simulink model "Casc_Filter_reva"  (Simulink 6.6)
settings: Solver=ode45  StartTime=0.0  StopTime=32768/sampling_freq  RelTol=1e-3
values from neighbouring files (symbols this model uses):
  filter_clk = sampling_freq*clk_mult    (= 375000000)    [Cascade_Taps_reva.m]    (also in Casecade_Taps.m)
  h_g = round(h_g*2^17)/2^17    [Cascade_Taps_reva.m]    (also in Casecade_Taps.m)
  h_k = round(h_k*2^17)/2^17    [Cascade_Taps_reva.m]    (also in Casecade_Taps.m)
  sampling_freq = 125e6    (= 125000000)    [Cascade_Taps_reva.m]    (also in Casecade_Taps.m)
undefined symbols (not defined in the file or in its folder): A, B, Fs, get, PCIN
libraries: xbsIndex_r4 x314, dspsnks4 x3, dspsrcs4 x2, simulink x2
(part 1 of 3)
settings Model: Creator=tbrimeye  LastModifiedBy=ericloew
settings DebuggingCC: SignalResolutionControl=TryResolveAllWithWarning  MultiTaskDSMMsg=warning  MultiTaskCondExecSysMsg=none
settings RTWCC: IncludeERTFirstTime=on

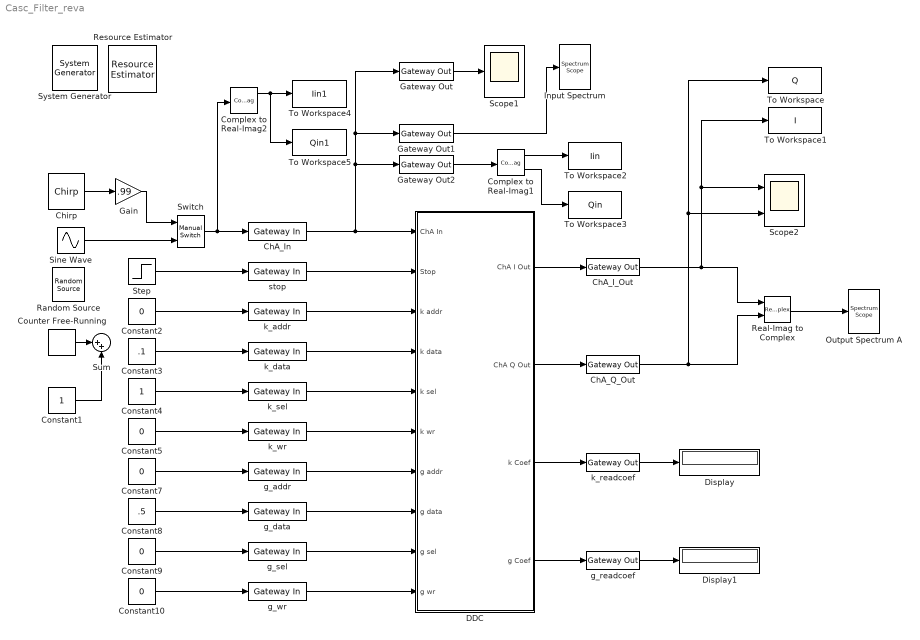
== system Casc_Filter_reva ==
  " System Generator" : xbsIndex_r4/ System Generator  Tag=genX  SystemSampleTime=-1  xilinxfamily=virtex4  part=xc4vsx55  speed=-10  package=ff1148  synthesis_tool=XST  directory=C:/GateFlow/7142_sig/4953_s142/xc4vsx55/Matlab/SysGen_Outputs  testbench=off  simulink_period=1/filter_clk  sysclk_period=(1/filter_clk)*1e9  incr_netlist=off  trim_vbits=Everywhere in SubSystem  dbl_ovrd=According to Block Masks  core_generation=According to Block Masks  run_coregen=off  deprecated_control=off  eval_field=0  block_type=sysgen
      settings: block_version=8.2
  ChA_I_Out : xbsIndex_r4/Gateway Out  hdl_port=on  timing_constraint=Data Rate  locs_specified=off  LOCs={}  block_type=gatewayout
      settings: infoedit="Gateway out block.  Converts Xilinx fixed point inputs into ouputs of type Simulink integer, double, or fixed point.<P><P>Hardware notes:  In hardware these blocks become top level output ports or are discarded, depending on how they are configured."  xl_area=[0 0 0 0 16 0 0]  block_version=8.2
  ChA_In : xbsIndex_r4/Gateway In  arith_type="Signed  (2's comp)"  n_bits=14  bin_pt=13  quantization="Round  (unbiased: +/- Inf)"  overflow=Saturate  period=1/sampling_freq  dbl_ovrd=off  timing_constraint=Data Rate  locs_specified=off  LOCs={}  block_type=gatewayin
      settings: infoedit="Gateway in block.  Converts inputs of type Simulink integer, double and fixed point to  Xilinx fixed point type.<P><P>Hardware notes:  In hardware these blocks become top level input ports."  xl_area=[0 0 0 0 14 0 0]  block_version=8.2
  ChA_Q_Out : xbsIndex_r4/Gateway Out  hdl_port=on  timing_constraint=Data Rate  locs_specified=off  LOCs={}  block_type=gatewayout
      settings: infoedit="Gateway out block.  Converts Xilinx fixed point inputs into ouputs of type Simulink integer, double, or fixed point.<P><P>Hardware notes:  In hardware these blocks become top level output ports or are discarded, depending on how they are configured."  xl_area=[0 0 0 0 16 0 0]  block_version=8.2
  Chirp : dspsrcs4/Chirp  sweep=Linear  mode=Unidirectional  f0=148.25e6  f1=164.25e6  t1=8192/sampling_freq  Tsweep=8192/sampling_freq  phase=pi/4  Ts=1/sampling_freq  spf=1  datatype=Double
  Complex to Real-Imag1 : ComplexToRealImag
  Complex to Real-Imag2 : ComplexToRealImag
  Constant1 : Constant
  Constant{2,5,7,9..10} (5 alike) : Constant  Value=0
  Constant3 : Constant  Value=.1
  Constant4 : Constant
  Constant8 : Constant  Value=.5
  Counter Free-Running : simulink/Sources/Counter Free-Running  SystemSampleTime=-1  NumBits=16  tsamp=1/sampling_freq
  DDC : Subsystem
  Display : Display
  Display1 : Display
  Gain : Gain  Gain=.99
  Gateway Out : xbsIndex_r4/Gateway Out  hdl_port=off  timing_constraint=None  locs_specified=off  LOCs={}  block_type=gatewayout
      settings: infoedit="Gateway out block.  Converts Xilinx fixed point inputs into ouputs of type Simulink integer, double, or fixed point.<P><P>Hardware notes:  In hardware these blocks become top level output ports or are discarded, depending on how they are configured."  block_version=8.2
  Gateway Out1 : xbsIndex_r4/Gateway Out  hdl_port=off  timing_constraint=None  locs_specified=off  LOCs={}  block_type=gatewayout
      settings: infoedit="Gateway out block.  Converts Xilinx fixed point inputs into ouputs of type Simulink integer, double, or fixed point.<P><P>Hardware notes:  In hardware these blocks become top level output ports or are discarded, depending on how they are configured."  block_version=8.2
  Gateway Out2 : xbsIndex_r4/Gateway Out  hdl_port=off  timing_constraint=None  locs_specified=off  LOCs={}  block_type=gatewayout
      settings: infoedit="Gateway out block.  Converts Xilinx fixed point inputs into ouputs of type Simulink integer, double, or fixed point.<P><P>Hardware notes:  In hardware these blocks become top level output ports or are discarded, depending on how they are configured."  block_version=8.2
  Input Spectrum : dspsnks4/Spectrum Scope  DialogController=dspdialog.SpectrumScope  DialogControllerArgs=DataTag2  SystemSampleTime=-1  ScopeProperties=on  Domain=Frequency  HorizSpan=1  UseBuffer=on  BufferSize=4096  Overlap=64  inpFftLenInherit=on  FFTlength=4096  numAvg=4  DisplayProperties=off  AxisGrid=on  Memory=off  FrameNumber=on  AxisLegend=off  AxisZoom=off  OpenScopeAtSimStart=on  OpenScopeImmediately=off  FigPos=get(0,'defaultfigureposition')  AxisProperties=off  XUnits=Hertz  XRange=[-Fs/2...Fs/2]  InheritXIncr=on  XIncr=1.0  XLabel=Samples  XLimit=Auto  YUnits=dB  XMax=1  XMin=0  YLabel=Magnitude-squared, dB  LineProperties=off  wintypeSpecScope=Boxcar  RsSpecScope=50  betaSpecScope=5  winsampSpecScope=Periodic
      settings: YMin=-38.4292198849576  YMax=29.4113653509126
  Output Spectrum A : dspsnks4/Spectrum Scope  DialogController=dspdialog.SpectrumScope  DialogControllerArgs=DataTag3  SystemSampleTime=-1  ScopeProperties=on  Domain=Frequency  HorizSpan=1  UseBuffer=on  BufferSize=1024  Overlap=64  inpFftLenInherit=on  FFTlength=1024  numAvg=1  DisplayProperties=off  AxisGrid=on  Memory=off  FrameNumber=on  AxisLegend=off  AxisZoom=off  OpenScopeAtSimStart=on  OpenScopeImmediately=off  FigPos=get(0,'defaultfigureposition')  AxisProperties=off  XUnits=Hertz  XRange=[-Fs/2...Fs/2]  InheritXIncr=on  XIncr=1.0  XLabel=Samples  XLimit=Auto  YUnits=dB  XMax=1  XMin=0  YLabel=Magnitude-squared, dB  LineProperties=off  wintypeSpecScope=Boxcar  RsSpecScope=50  betaSpecScope=5  winsampSpecScope=Symmetric
      settings: YMin=-135.913616439453  YMax=3.76850779494313
  Random Source : dspsrcs4/Random Source  SrcType=Uniform  NormMethod=Ziggurat  CltLength=12  MinVal=-1  MaxVal=1  MeanVal=0  VarVal=1  RepMode=Not repeatable  rawSeed=1  IsInherit=off  SampMode=Discrete  SampTime=1/sampling_freq  SampFrame=1  DataType=Double  OutComplex=Real
  Real-Imag to Complex : RealImagToComplex
  Resource Estimator : xbsIndex_r4/Resource Estimator  Tag=resEstTag  Slices=925  FFs=1405  BRAMs=7  LUTs=1104  IOBs=133  EBMs=14  TBUFs=0  xl_use_estimator_area=off  est_options=Post Map  xl_estimator_area=[1915 2342 0 3405 33 4 0]  block_type=resource_estimator
      settings: AttributesFormatString=Resource\nEstimator  block_version=8.2
  Scope1 : Scope
      settings: SaveName=ScopeData2
  Scope2 : Scope  NumInputPorts=2
      settings: YMin=-5~-5  YMax=5~5  SaveName=ScopeData4
  Sine Wave : Sin  Amplitude=.99  Frequency=2*pi*156.75e6  SampleTime=1/sampling_freq
  Step : Step  Time=00/filter_clk  Before=1  After=0  SampleTime=1/filter_clk
  Sum : Sum  Inputs=|++
  Switch : simulink/Signal Routing/Manual Switch  SystemSampleTime=-1  sw=1  action=0  varsize=off
  To Workspace : ToWorkspace  VariableName=Q  SampleTime=-1  SaveFormat=Array
  To Workspace1 : ToWorkspace  VariableName=I  SampleTime=-1  SaveFormat=Array
  To Workspace2 : ToWorkspace  VariableName=Iin  SampleTime=-1  SaveFormat=Array
  To Workspace3 : ToWorkspace  VariableName=Qin  SampleTime=-1  SaveFormat=Array
  To Workspace4 : ToWorkspace  VariableName=Iin1  SampleTime=-1  SaveFormat=Array
  To Workspace5 : ToWorkspace  VariableName=Qin1  SampleTime=-1  SaveFormat=Array
  g_addr : xbsIndex_r4/Gateway In  arith_type=Unsigned  n_bits=4  bin_pt=0  quantization="Round  (unbiased: +/- Inf)"  overflow=Saturate  period=1/sampling_freq  dbl_ovrd=off  timing_constraint=None  locs_specified=off  LOCs={}  block_type=gatewayin
      settings: infoedit="Gateway in block.  Converts inputs of type Simulink integer, double and fixed point to  Xilinx fixed point type.<P><P>Hardware notes:  In hardware these blocks become top level input ports."  xl_area=[0 0 0 0 4 0 0]  block_version=VER_STRING_GOES_HERE
  g_data : xbsIndex_r4/Gateway In  arith_type="Signed  (2's comp)"  n_bits=18  bin_pt=17  quantization="Round  (unbiased: +/- Inf)"  overflow=Saturate  period=1/sampling_freq  dbl_ovrd=off  timing_constraint=None  locs_specified=off  LOCs={}  block_type=gatewayin
      settings: infoedit="Gateway in block.  Converts inputs of type Simulink integer, double and fixed point to  Xilinx fixed point type.<P><P>Hardware notes:  In hardware these blocks become top level input ports."  xl_area=[0 0 0 0 18 0 0]  block_version=VER_STRING_GOES_HERE
  g_readcoef : xbsIndex_r4/Gateway Out  hdl_port=on  timing_constraint=Data Rate  locs_specified=off  LOCs={}  block_type=gatewayout
      settings: infoedit="Gateway out block.  Converts Xilinx fixed point inputs into ouputs of type Simulink integer, double, or fixed point.<P><P>Hardware notes:  In hardware these blocks become top level output ports or are discarded, depending on how they are configured."  xl_area=[0 0 0 0 18 0 0]  block_version=VER_STRING_GOES_HERE
  g_sel : xbsIndex_r4/Gateway In  arith_type=Unsigned  n_bits=2  bin_pt=0  quantization="Round  (unbiased: +/- Inf)"  overflow=Saturate  period=1/sampling_freq  dbl_ovrd=off  timing_constraint=None  locs_specified=off  LOCs={}  block_type=gatewayin
      settings: infoedit="Gateway in block.  Converts inputs of type Simulink integer, double and fixed point to  Xilinx fixed point type.<P><P>Hardware notes:  In hardware these blocks become top level input ports."  xl_area=[0 0 0 0 2 0 0]  block_version=VER_STRING_GOES_HERE
  g_wr : xbsIndex_r4/Gateway In  arith_type=Boolean  n_bits=4  bin_pt=0  quantization="Round  (unbiased: +/- Inf)"  overflow=Saturate  period=1/sampling_freq  dbl_ovrd=off  timing_constraint=None  locs_specified=off  LOCs={}  block_type=gatewayin
      settings: infoedit="Gateway in block.  Converts inputs of type Simulink integer, double and fixed point to  Xilinx fixed point type.<P><P>Hardware notes:  In hardware these blocks become top level input ports."  xl_area=[0 0 0 0 1 0 0]  block_version=VER_STRING_GOES_HERE
  k_addr : xbsIndex_r4/Gateway In  arith_type=Unsigned  n_bits=4  bin_pt=0  quantization="Round  (unbiased: +/- Inf)"  overflow=Saturate  period=1/sampling_freq  dbl_ovrd=off  timing_constraint=None  locs_specified=off  LOCs={}  block_type=gatewayin
      settings: infoedit="Gateway in block.  Converts inputs of type Simulink integer, double and fixed point to  Xilinx fixed point type.<P><P>Hardware notes:  In hardware these blocks become top level input ports."  xl_area=[0 0 0 0 4 0 0]  block_version=VER_STRING_GOES_HERE
  k_data : xbsIndex_r4/Gateway In  arith_type="Signed  (2's comp)"  n_bits=18  bin_pt=17  quantization="Round  (unbiased: +/- Inf)"  overflow=Saturate  period=1/sampling_freq  dbl_ovrd=off  timing_constraint=None  locs_specified=off  LOCs={}  block_type=gatewayin
      settings: infoedit="Gateway in block.  Converts inputs of type Simulink integer, double and fixed point to  Xilinx fixed point type.<P><P>Hardware notes:  In hardware these blocks become top level input ports."  xl_area=[0 0 0 0 18 0 0]  block_version=VER_STRING_GOES_HERE
  k_readcoef : xbsIndex_r4/Gateway Out  hdl_port=on  timing_constraint=Data Rate  locs_specified=off  LOCs={}  block_type=gatewayout
      settings: infoedit="Gateway out block.  Converts Xilinx fixed point inputs into ouputs of type Simulink integer, double, or fixed point.<P><P>Hardware notes:  In hardware these blocks become top level output ports or are discarded, depending on how they are configured."  xl_area=[0 0 0 0 18 0 0]  block_version=VER_STRING_GOES_HERE
  k_sel : xbsIndex_r4/Gateway In  arith_type=Unsigned  n_bits=3  bin_pt=0  quantization="Round  (unbiased: +/- Inf)"  overflow=Saturate  period=1/sampling_freq  dbl_ovrd=off  timing_constraint=None  locs_specified=off  LOCs={}  block_type=gatewayin
      settings: infoedit="Gateway in block.  Converts inputs of type Simulink integer, double and fixed point to  Xilinx fixed point type.<P><P>Hardware notes:  In hardware these blocks become top level input ports."  xl_area=[0 0 0 0 2 0 0]  block_version=VER_STRING_GOES_HERE
  k_wr : xbsIndex_r4/Gateway In  arith_type=Boolean  n_bits=4  bin_pt=0  quantization="Round  (unbiased: +/- Inf)"  overflow=Saturate  period=1/sampling_freq  dbl_ovrd=off  timing_constraint=None  locs_specified=off  LOCs={}  block_type=gatewayin
      settings: infoedit="Gateway in block.  Converts inputs of type Simulink integer, double and fixed point to  Xilinx fixed point type.<P><P>Hardware notes:  In hardware these blocks become top level input ports."  xl_area=[0 0 0 0 1 0 0]  block_version=VER_STRING_GOES_HERE
  stop : xbsIndex_r4/Gateway In  arith_type=Unsigned  n_bits=1  bin_pt=0  quantization="Round  (unbiased: +/- Inf)"  overflow=Saturate  period=1/sampling_freq  dbl_ovrd=off  timing_constraint=Data Rate  locs_specified=off  LOCs={}  block_type=gatewayin
      settings: infoedit="Gateway in block.  Converts inputs of type Simulink integer, double and fixed point to  Xilinx fixed point type.<P><P>Hardware notes:  In hardware these blocks become top level input ports."  xl_area=[0 0 0 0 1 0 0]  block_version=VER_STRING_GOES_HERE
  wires:
  Chirp/1 -> Gain/1
  ChA_In/1 -> DDC/1(ChA In), Gateway Out1/1, Gateway Out/1, Gateway Out2/1
  Real-Imag to Complex/1 -> Output Spectrum A/1
  Switch/1 -> ChA_In/1, Complex to Real-Imag2/1
  ChA_I_Out/1 -> Real-Imag to Complex/1, Scope2/1, To Workspace1/1
  ChA_Q_Out/1 -> Real-Imag to Complex/2, Scope2/2, To Workspace/1
  k_sel/1 -> DDC/5(k sel)
  k_addr/1 -> DDC/3(k addr)
  k_data/1 -> DDC/4(k data)
  k_wr/1 -> DDC/6(k wr)
  DDC/3(k Coef) -> k_readcoef/1
  Constant2/1 -> k_addr/1
  Constant3/1 -> k_data/1
  Constant4/1 -> k_sel/1
  Constant5/1 -> k_wr/1
  k_readcoef/1 -> Display/1
  g_readcoef/1 -> Display1/1
  DDC/4(g Coef) -> g_readcoef/1
  g_addr/1 -> DDC/7(g addr)
  g_data/1 -> DDC/8(g data)
  g_sel/1 -> DDC/9(g sel)
  g_wr/1 -> DDC/10(g wr)
  Constant7/1 -> g_addr/1
  Constant8/1 -> g_data/1
  Constant9/1 -> g_sel/1
  Constant10/1 -> g_wr/1
  DDC/1(ChA I Out) -> ChA_I_Out/1
  DDC/2(ChA Q Out) -> ChA_Q_Out/1
  stop/1 -> DDC/2(Stop)
  Gateway Out/1 -> Scope1/1
  Gateway Out1/1 -> Input Spectrum/1
  Gain/1 -> Switch/1
  Gateway Out2/1 -> Complex to Real-Imag1/1
  Complex to Real-Imag2/1 -> To Workspace4/1, To Workspace5/1
  Step/1 -> stop/1
  Counter Free-Running/1 -> Sum/1
  Constant1/1 -> Sum/2
  Complex to Real-Imag1/1 -> To Workspace2/1
  Complex to Real-Imag1/2 -> To Workspace3/1
  Sine Wave/1 -> Switch/2

== system Casc_Filter_reva/DDC ==
  ChA In : Inport
  Stop : Inport  Port=2
  k addr : Inport  Port=3
  k data : Inport  Port=4
  k sel : Inport  Port=5
  k wr : Inport  Port=6
  g addr : Inport  Port=7
  g data : Inport  Port=8
  g sel : Inport  Port=9
  g wr : Inport  Port=10
  Coefficients : Subsystem
  Count Generator : Subsystem
  DDC A : Subsystem
  Display : Display
  ChA I Out : Outport
  ChA Q Out : Outport  Port=2
  k Coef : Outport  Port=3
  g Coef : Outport  Port=4
  wires:
  Count Generator/1(Count) -> Coefficients/1(Counter), DDC A/1(Counter)
  Coefficients/1(k_Coef0) -> DDC A/4(k_Coef0)
  Coefficients/2(k_Coef1) -> DDC A/5(k_Coef1)
  Coefficients/3(k_Coef2) -> DDC A/6(k_Coef2)
  Coefficients/4(k_Coef3) -> DDC A/7(k_Coef3)
  Count Generator/2(Invert Count) -> DDC A/2(Counter Inv)
  Coefficients/5(g_Coef0) -> DDC A/12(g_Coef0), Display/1
  Coefficients/10(g_Coef1) -> DDC A/13(g_Coef1)
  Coefficients/11(g_Coef2) -> DDC A/14(g_Coef2)
  ChA In/1 -> DDC A/3(Data In Ch A)
  Stop/1 -> Coefficients/2(Stop), Count Generator/1(Reset)
  k addr/1 -> Coefficients/3(k_addr)
  k data/1 -> Coefficients/4(k_data)
  k sel/1 -> Coefficients/5(k_sel)
  k wr/1 -> Coefficients/6(k_wr)
  g addr/1 -> Coefficients/7(g_addr)
  g data/1 -> Coefficients/8(g_data)
  Coefficients/12(k_CoefRead) -> k Coef/1
  g sel/1 -> Coefficients/9(g_sel)
  g wr/1 -> Coefficients/10(g_wr)
  Coefficients/13(g_CoefRead) -> g Coef/1
  DDC A/1(I Out) -> ChA I Out/1
  DDC A/2(Q Out) -> ChA Q Out/1
  Coefficients/6(k_Coef4) -> DDC A/8(k_Coef4)
  Coefficients/7(k_Coef5) -> DDC A/9(k_Coef5)
  Coefficients/8(k_Coef6) -> DDC A/10(k_Coef6)
  Coefficients/9(k_Coef7) -> DDC A/11(k_Coef7)

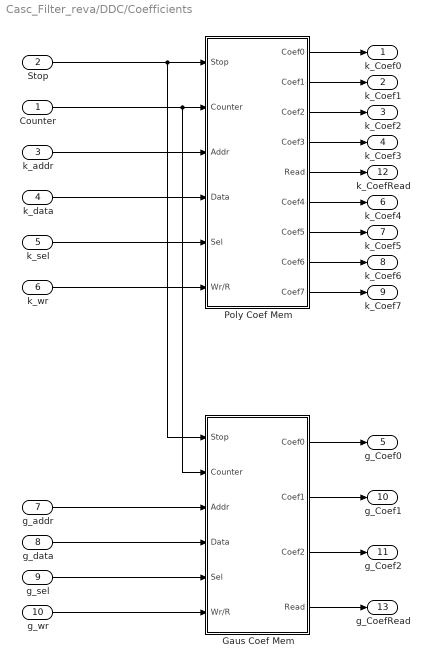
== system Casc_Filter_reva/DDC/Coefficients ==
  Counter : Inport
  Stop : Inport  Port=2
  k_addr : Inport  Port=3
  k_data : Inport  Port=4
  k_sel : Inport  Port=5
  k_wr : Inport  Port=6
  g_addr : Inport  Port=7
  g_data : Inport  Port=8
  g_sel : Inport  Port=9
  g_wr : Inport  Port=10
  Gaus Coef Mem : Subsystem
  Poly Coef Mem : Subsystem
  k_Coef0 : Outport
  k_Coef1 : Outport  Port=2
  k_Coef2 : Outport  Port=3
  k_Coef3 : Outport  Port=4
  g_Coef0 : Outport  Port=5
  k_Coef4 : Outport  Port=6
  k_Coef5 : Outport  Port=7
  k_Coef6 : Outport  Port=8
  k_Coef7 : Outport  Port=9
  g_Coef1 : Outport  Port=10
  g_Coef2 : Outport  Port=11
  k_CoefRead : Outport  Port=12
  g_CoefRead : Outport  Port=13
  wires:
  Stop/1 -> Gaus Coef Mem/1(Stop), Poly Coef Mem/1(Stop)
  Counter/1 -> Poly Coef Mem/2(Counter), Gaus Coef Mem/2(Counter)
  Poly Coef Mem/1(Coef0) -> k_Coef0/1
  Poly Coef Mem/2(Coef1) -> k_Coef1/1
  k_addr/1 -> Poly Coef Mem/3(Addr)
  Poly Coef Mem/3(Coef2) -> k_Coef2/1
  k_data/1 -> Poly Coef Mem/4(Data)
  Poly Coef Mem/4(Coef3) -> k_Coef3/1
  k_sel/1 -> Poly Coef Mem/5(Sel)
  Poly Coef Mem/5(Read) -> k_CoefRead/1
  k_wr/1 -> Poly Coef Mem/6(Wr/R)
  Gaus Coef Mem/1(Coef0) -> g_Coef0/1
  Gaus Coef Mem/2(Coef1) -> g_Coef1/1
  g_addr/1 -> Gaus Coef Mem/3(Addr)
  g_data/1 -> Gaus Coef Mem/4(Data)
  Gaus Coef Mem/3(Coef2) -> g_Coef2/1
  g_sel/1 -> Gaus Coef Mem/5(Sel)
  Gaus Coef Mem/4(Read) -> g_CoefRead/1
  g_wr/1 -> Gaus Coef Mem/6(Wr/R)
  Poly Coef Mem/6(Coef4) -> k_Coef4/1
  Poly Coef Mem/7(Coef5) -> k_Coef5/1
  Poly Coef Mem/8(Coef6) -> k_Coef6/1
  Poly Coef Mem/9(Coef7) -> k_Coef7/1

== system Casc_Filter_reva/DDC/Count Generator ==
  Reset : Inport
  AddSub : xbsIndex_r4/AddSub  mode=Subtraction  use_carryin=off  use_carryout=off  en=off  latency=0  precision=User Defined  arith_type=Unsigned  n_bits=3  bin_pt=0  quantization=Truncate  overflow=Wrap  dbl_ovrd=off  use_behavioral_HDL=off  pipelined=off  use_rpm=on  block_type=addsub
      settings: block_version=9.2.01
  Constant : xbsIndex_r4/Constant  arith_type=Unsigned  const=7  n_bits=4  bin_pt=0  explicit_period=off  period=1  equ=P=C  opselect=C  inp2=PCIN>>17  opr=+  inp1=P  carry=CIN  dbl_ovrd=off  block_type=constant
      settings: block_version=9.2.01
  Convert : xbsIndex_r4/Convert  arith_type=Boolean  n_bits=16  bin_pt=14  quantization=Truncate  overflow=Wrap  latency=0  dbl_ovrd=off  pipeline=off  block_type=convert
      settings: block_version=9.2.01
  Counter : xbsIndex_r4/Counter  cnt_type=Count Limited  cnt_to=7  operation=Up  start_count=0  cnt_by_val=1  arith_type=Unsigned  n_bits=3  bin_pt=0  load_pin=off  rst=on  en=off  explicit_period=on  period=1/filter_clk  dbl_ovrd=off  use_behavioral_HDL=off  use_rpm=off  block_type=counter
      settings: block_version=8.2
  Count : Outport
  Invert Count : Outport  Port=2
  wires:
  Counter/1 -> AddSub/2, Count/1
  Constant/1 -> AddSub/1
  Convert/1 -> Counter/1
  Reset/1 -> Convert/1
  AddSub/1 -> Invert Count/1

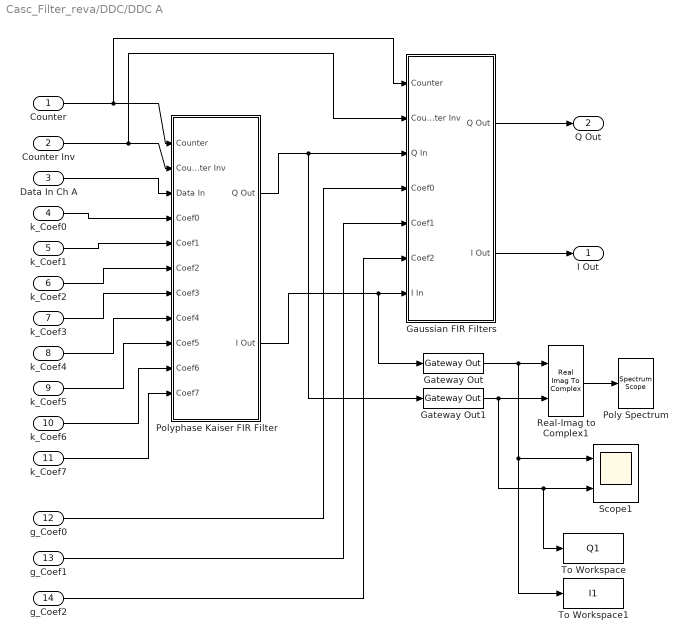
== system Casc_Filter_reva/DDC/DDC A ==
  Counter : Inport
  Counter Inv : Inport  Port=2
  Data In Ch A : Inport  Port=3
  k_Coef0 : Inport  Port=4
  k_Coef1 : Inport  Port=5
  k_Coef2 : Inport  Port=6
  k_Coef3 : Inport  Port=7
  k_Coef4 : Inport  Port=8
  k_Coef5 : Inport  Port=9
  k_Coef6 : Inport  Port=10
  k_Coef7 : Inport  Port=11
  g_Coef0 : Inport  Port=12
  g_Coef1 : Inport  Port=13
  g_Coef2 : Inport  Port=14
  Gateway Out : xbsIndex_r4/Gateway Out  hdl_port=off  timing_constraint=None  locs_specified=off  LOCs={}  block_type=gatewayout
      settings: infoedit="Gateway out block.  Converts Xilinx fixed point inputs into ouputs of type Simulink integer, double, or fixed point.<P><P>Hardware notes:  In hardware these blocks become top level output ports or are discarded, depending on how they are configured."  block_version=8.2
  Gateway Out1 : xbsIndex_r4/Gateway Out  hdl_port=off  timing_constraint=None  locs_specified=off  LOCs={}  block_type=gatewayout
      settings: infoedit="Gateway out block.  Converts Xilinx fixed point inputs into ouputs of type Simulink integer, double, or fixed point.<P><P>Hardware notes:  In hardware these blocks become top level output ports or are discarded, depending on how they are configured."  block_version=8.2
  Gaussian FIR Filters : Subsystem
  Poly Spectrum : dspsnks4/Spectrum Scope  DialogController=dspdialog.SpectrumScope  DialogControllerArgs=DataTag1  SystemSampleTime=-1  ScopeProperties=on  Domain=Frequency  HorizSpan=1  UseBuffer=on  BufferSize=1024  Overlap=64  inpFftLenInherit=on  FFTlength=1024  numAvg=1  DisplayProperties=off  AxisGrid=on  Memory=off  FrameNumber=on  AxisLegend=off  AxisZoom=off  OpenScopeAtSimStart=on  OpenScopeImmediately=off  FigPos=get(0,'defaultfigureposition')  AxisProperties=off  XUnits=Hertz  XRange=[-Fs/2...Fs/2]  InheritXIncr=on  XIncr=1.0  XLabel=Samples  XLimit=Auto  YUnits=dB  XMax=1  XMin=0  YLabel=Magnitude-squared, dB  LineProperties=off  wintypeSpecScope=Boxcar  RsSpecScope=50  betaSpecScope=5  winsampSpecScope=Periodic
      settings: YMin=-87.1539985326234  YMax=2.74033893845064
  Polyphase Kaiser FIR Filter : Subsystem
  Real-Imag to Complex1 : RealImagToComplex
  Scope1 : Scope  NumInputPorts=2
      settings: YMin=-5~-5  YMax=5~5  SaveName=ScopeData3
  To Workspace : ToWorkspace  VariableName=Q1  SampleTime=-1  SaveFormat=Array
  To Workspace1 : ToWorkspace  VariableName=I1  SampleTime=-1  SaveFormat=Array
  I Out : Outport
  Q Out : Outport  Port=2
  wires:
  Counter Inv/1 -> Polyphase Kaiser FIR Filter/2(Counter Inv), Gaussian FIR Filters/2(Counter Inv)
  Real-Imag to Complex1/1 -> Poly Spectrum/1
  Counter/1 -> Polyphase Kaiser FIR Filter/1(Counter), Gaussian FIR Filters/1(Counter)
  Gaussian FIR Filters/1(Q Out) -> Q Out/1
  Data In Ch A/1 -> Polyphase Kaiser FIR Filter/3(Data In)
  k_Coef0/1 -> Polyphase Kaiser FIR Filter/4(Coef0)
  Gaussian FIR Filters/2(I Out) -> I Out/1
  k_Coef1/1 -> Polyphase Kaiser FIR Filter/5(Coef1)
  k_Coef2/1 -> Polyphase Kaiser FIR Filter/6(Coef2)
  Polyphase Kaiser FIR Filter/1(Q Out) -> Gaussian FIR Filters/3(Q In), Gateway Out1/1
  Polyphase Kaiser FIR Filter/2(I Out) -> Gaussian FIR Filters/7(I In), Gateway Out/1
  g_Coef0/1 -> Gaussian FIR Filters/4(Coef0)
  g_Coef1/1 -> Gaussian FIR Filters/5(Coef1)
  g_Coef2/1 -> Gaussian FIR Filters/6(Coef2)
  Gateway Out/1 -> Real-Imag to Complex1/1, Scope1/1, To Workspace1/1
  Gateway Out1/1 -> Real-Imag to Complex1/2, To Workspace/1, Scope1/2
  k_Coef4/1 -> Polyphase Kaiser FIR Filter/8(Coef4)
  k_Coef6/1 -> Polyphase Kaiser FIR Filter/10(Coef6)
  k_Coef7/1 -> Polyphase Kaiser FIR Filter/11(Coef7)
  k_Coef3/1 -> Polyphase Kaiser FIR Filter/7(Coef3)
  k_Coef5/1 -> Polyphase Kaiser FIR Filter/9(Coef5)

== system Casc_Filter_reva/DDC/Coefficients/Gaus Coef Mem ==
  Stop : Inport
  Counter : Inport  Port=2
  Addr : Inport  Port=3
  Data : Inport  Port=4
  Sel : Inport  Port=5
  Wr/R : Inport  Port=6
  Mux : xbsIndex_r4/Mux  inputs=2  en=off  latency=1  precision=Full  arith_type=Unsigned  n_bits=16  bin_pt=14  quantization=Truncate  overflow=Wrap  dbl_ovrd=off  block_type=mux
      settings: xl_area=[2 0 0 4 0 0 0]  block_version=VER_STRING_GOES_HERE
  Mux1 : xbsIndex_r4/Mux  inputs=3  en=on  latency=1  precision=Full  arith_type=Unsigned  n_bits=16  bin_pt=14  quantization=Truncate  overflow=Wrap  dbl_ovrd=off  block_type=mux
      settings: xl_area=[18 18 0 36 0 0 0]  block_version=VER_STRING_GOES_HERE
  Select Decoder : Subsystem
  Single Port RAM : xbsIndex_r4/Single Port RAM  depth=16  initVector=[h_g(1:8),0,0,0,0,0,0,0,0]  distributed_mem=Block RAM  write_mode=No Read On Write  rst=off  init_reg=0  en=off  latency=7  dbl_ovrd=off  optimize=Area  use_rpm=off  block_type=spram
      settings: xl_area=[18 0 0 36 0 0 0]  block_version=8.2
  Single Port RAM1 : xbsIndex_r4/Single Port RAM  depth=16  initVector=[h_g(9:16),0,0,0,0,0,0,0,0]  distributed_mem=Block RAM  write_mode=No Read On Write  rst=off  init_reg=0  en=off  latency=7  dbl_ovrd=off  optimize=Area  use_rpm=off  block_type=spram
      settings: xl_area=[18 0 0 36 0 0 0]  block_version=8.2
  Single Port RAM2 : xbsIndex_r4/Single Port RAM  depth=16  initVector=[h_g(17:24),0,0,0,0,0,0,0,0]  distributed_mem=Block RAM  write_mode=No Read On Write  rst=off  init_reg=0  en=off  latency=7  dbl_ovrd=off  optimize=Area  use_rpm=off  block_type=spram
      settings: xl_area=[18 0 0 36 0 0 0]  block_version=8.2
  Coef0 : Outport
  Coef1 : Outport  Port=2
  Coef2 : Outport  Port=3
  Read : Outport  Port=4
  wires:
  Data/1 -> Single Port RAM1/2, Single Port RAM2/2, Single Port RAM/2
  Single Port RAM/1 -> Mux1/2, Coef0/1
  Single Port RAM1/1 -> Mux1/3, Coef1/1
  Single Port RAM2/1 -> Mux1/4, Coef2/1
  Stop/1 -> Mux/1, Select Decoder/1(Run/Stop)
  Mux/1 -> Single Port RAM/1, Single Port RAM1/1, Single Port RAM2/1
  Mux1/1 -> Read/1
  Counter/1 -> Mux/2
  Addr/1 -> Mux/3
  Sel/1 -> Select Decoder/3(Sel), Mux1/1
  Select Decoder/2(Wr0) -> Single Port RAM/3
  Select Decoder/3(Wr1) -> Single Port RAM1/3
  Select Decoder/4(Wr2) -> Single Port RAM2/3
  Wr/R/1 -> Select Decoder/2(Wr/R)
  Select Decoder/1(R_En) -> Mux1/5

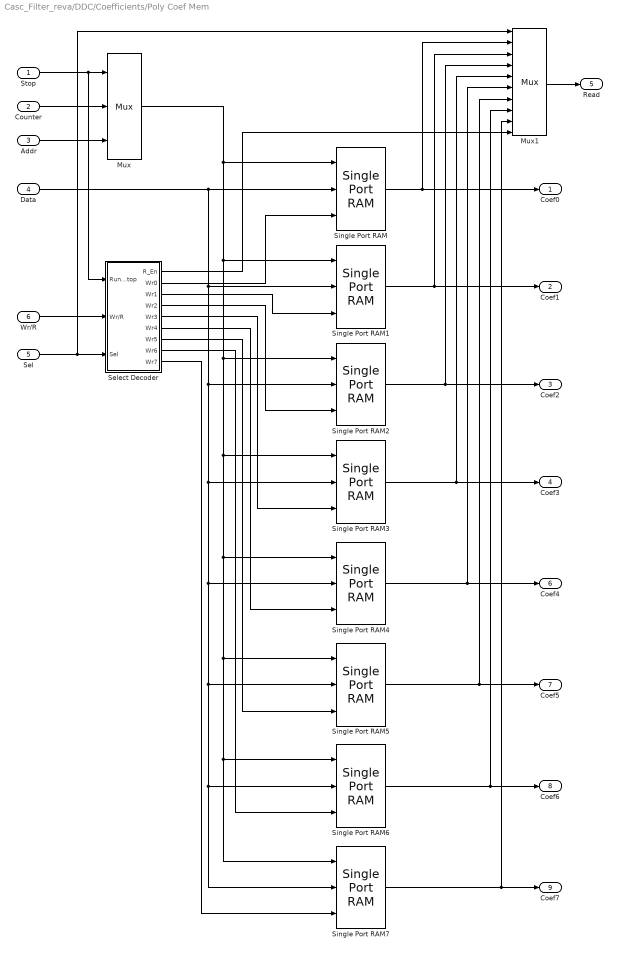
== system Casc_Filter_reva/DDC/Coefficients/Poly Coef Mem ==
  Stop : Inport
  Counter : Inport  Port=2
  Addr : Inport  Port=3
  Data : Inport  Port=4
  Sel : Inport  Port=5
  Wr/R : Inport  Port=6
  Mux : xbsIndex_r4/Mux  inputs=2  en=off  latency=1  precision=Full  arith_type=Unsigned  n_bits=16  bin_pt=14  quantization=Truncate  overflow=Wrap  dbl_ovrd=off  block_type=mux
      settings: xl_area=[2 0 0 4 0 0 0]  block_version=VER_STRING_GOES_HERE
  Mux1 : xbsIndex_r4/Mux  inputs=8  en=on  latency=1  precision=Full  arith_type=Unsigned  n_bits=16  bin_pt=14  quantization=Truncate  overflow=Wrap  dbl_ovrd=off  block_type=mux
      settings: xl_area=[18 18 0 36 0 0 0]  block_version=VER_STRING_GOES_HERE
  Select Decoder : Subsystem
  Single Port RAM : xbsIndex_r4/Single Port RAM  depth=16  initVector=[h_k(1:8:64),0,0,0,0,0,0,0,0]  distributed_mem=Block RAM  write_mode=No Read On Write  rst=off  init_reg=0  en=off  latency=7  dbl_ovrd=off  optimize=Area  use_rpm=off  block_type=spram
      settings: xl_area=[18 0 0 36 0 0 0]  block_version=8.2
  Single Port RAM1 : xbsIndex_r4/Single Port RAM  depth=16  initVector=[h_k(2:8:64),0,0,0,0,0,0,0,0]  distributed_mem=Block RAM  write_mode=No Read On Write  rst=off  init_reg=0  en=off  latency=7  dbl_ovrd=off  optimize=Area  use_rpm=off  block_type=spram
      settings: xl_area=[18 0 0 36 0 0 0]  block_version=8.2
  Single Port RAM2 : xbsIndex_r4/Single Port RAM  depth=16  initVector=[h_k(3:8:64),0,0,0,0,0,0,0,0]  distributed_mem=Block RAM  write_mode=No Read On Write  rst=off  init_reg=0  en=off  latency=7  dbl_ovrd=off  optimize=Area  use_rpm=off  block_type=spram
      settings: xl_area=[18 0 0 36 0 0 0]  block_version=8.2
  Single Port RAM3 : xbsIndex_r4/Single Port RAM  depth=16  initVector=[h_k(4:8:64),0,0,0,0,0,0,0,0]  distributed_mem=Block RAM  write_mode=No Read On Write  rst=off  init_reg=0  en=off  latency=7  dbl_ovrd=off  optimize=Area  use_rpm=off  block_type=spram
      settings: xl_area=[18 0 0 36 0 0 0]  block_version=8.2
  Single Port RAM4 : xbsIndex_r4/Single Port RAM  depth=16  initVector=[h_k(5:8:64),0,0,0,0,0,0,0,0]  distributed_mem=Block RAM  write_mode=No Read On Write  rst=off  init_reg=0  en=off  latency=7  dbl_ovrd=off  optimize=Area  use_rpm=off  block_type=spram
      settings: xl_area=[18 0 0 36 0 0 0]  block_version=8.2
  Single Port RAM5 : xbsIndex_r4/Single Port RAM  depth=16  initVector=[h_k(6:8:64),0,0,0,0,0,0,0,0]  distributed_mem=Block RAM  write_mode=No Read On Write  rst=off  init_reg=0  en=off  latency=7  dbl_ovrd=off  optimize=Area  use_rpm=off  block_type=spram
      settings: xl_area=[18 0 0 36 0 0 0]  block_version=8.2
  Single Port RAM6 : xbsIndex_r4/Single Port RAM  depth=16  initVector=[h_k(7:8:64),0,0,0,0,0,0,0,0]  distributed_mem=Block RAM  write_mode=No Read On Write  rst=off  init_reg=0  en=off  latency=7  dbl_ovrd=off  optimize=Area  use_rpm=off  block_type=spram
      settings: xl_area=[18 0 0 36 0 0 0]  block_version=8.2
  Single Port RAM7 : xbsIndex_r4/Single Port RAM  depth=16  initVector=[h_k(8:8:64),0,0,0,0,0,0,0,0]  distributed_mem=Block RAM  write_mode=No Read On Write  rst=off  init_reg=0  en=off  latency=7  dbl_ovrd=off  optimize=Area  use_rpm=off  block_type=spram
      settings: xl_area=[18 0 0 36 0 0 0]  block_version=8.2
  Coef0 : Outport
  Coef1 : Outport  Port=2
  Coef2 : Outport  Port=3
  Coef3 : Outport  Port=4
  Read : Outport  Port=5
  Coef4 : Outport  Port=6
  Coef5 : Outport  Port=7
  Coef6 : Outport  Port=8
  Coef7 : Outport  Port=9
  wires:
  Data/1 -> Single Port RAM2/2, Single Port RAM3/2, Single Port RAM4/2, Single Port RAM5/2, Single Port RAM6/2, Single Port RAM7/2, Single Port RAM1/2, Single Port RAM/2
  Single Port RAM/1 -> Mux1/2, Coef0/1
  Single Port RAM1/1 -> Mux1/3, Coef1/1
  Single Port RAM2/1 -> Mux1/4, Coef2/1
  Single Port RAM3/1 -> Mux1/5, Coef3/1
  Stop/1 -> Mux/1, Select Decoder/1(Run/Stop)
  Mux/1 -> Single Port RAM1/1, Single Port RAM2/1, Single Port RAM3/1, Single Port RAM4/1, Single Port RAM5/1, Single Port RAM6/1, Single Port RAM7/1, Single Port RAM/1
  Mux1/1 -> Read/1
  Counter/1 -> Mux/2
  Addr/1 -> Mux/3
  Sel/1 -> Select Decoder/3(Sel), Mux1/1
  Wr/R/1 -> Select Decoder/2(Wr/R)
  Select Decoder/2(Wr0) -> Single Port RAM/3
  Select Decoder/3(Wr1) -> Single Port RAM1/3
  Select Decoder/4(Wr2) -> Single Port RAM2/3
  Select Decoder/5(Wr3) -> Single Port RAM3/3
  Select Decoder/1(R_En) -> Mux1/10
  Single Port RAM4/1 -> Coef4/1, Mux1/6
  Single Port RAM5/1 -> Coef5/1, Mux1/7
  Single Port RAM6/1 -> Coef6/1, Mux1/8
  Single Port RAM7/1 -> Coef7/1, Mux1/9
  Select Decoder/6(Wr4) -> Single Port RAM4/3
  Select Decoder/7(Wr5) -> Single Port RAM5/3
  Select Decoder/8(Wr6) -> Single Port RAM6/3
  Select Decoder/9(Wr7) -> Single Port RAM7/3

== system Casc_Filter_reva/DDC/DDC A/Gaussian FIR Filters ==
  Counter : Inport
  Counter Inv : Inport  Port=2
  Q In : Inport  Port=3
  Coef0 : Inport  Port=4
  Coef1 : Inport  Port=5
  Coef2 : Inport  Port=6
  I In : Inport  Port=7
  Gaussian FIR Filter : Subsystem
  Gaussian FIR Filter1 : Subsystem
  Q Out : Outport
  I Out : Outport  Port=2
  wires:
  Counter/1 -> Gaussian FIR Filter/1(Counter), Gaussian FIR Filter1/1(Counter)
  Counter Inv/1 -> Gaussian FIR Filter/2(Counter Inv), Gaussian FIR Filter1/2(Counter Inv)
  Q In/1 -> Gaussian FIR Filter/3(Data In)
  I In/1 -> Gaussian FIR Filter1/3(Data In)
  Gaussian FIR Filter/1(Data Out) -> Q Out/1
  Gaussian FIR Filter1/1(Data Out) -> I Out/1
  Coef0/1 -> Gaussian FIR Filter/4(Coef0), Gaussian FIR Filter1/4(Coef0)
  Coef1/1 -> Gaussian FIR Filter/5(Coef1), Gaussian FIR Filter1/5(Coef1)
  Coef2/1 -> Gaussian FIR Filter/6(Coef2), Gaussian FIR Filter1/6(Coef2)

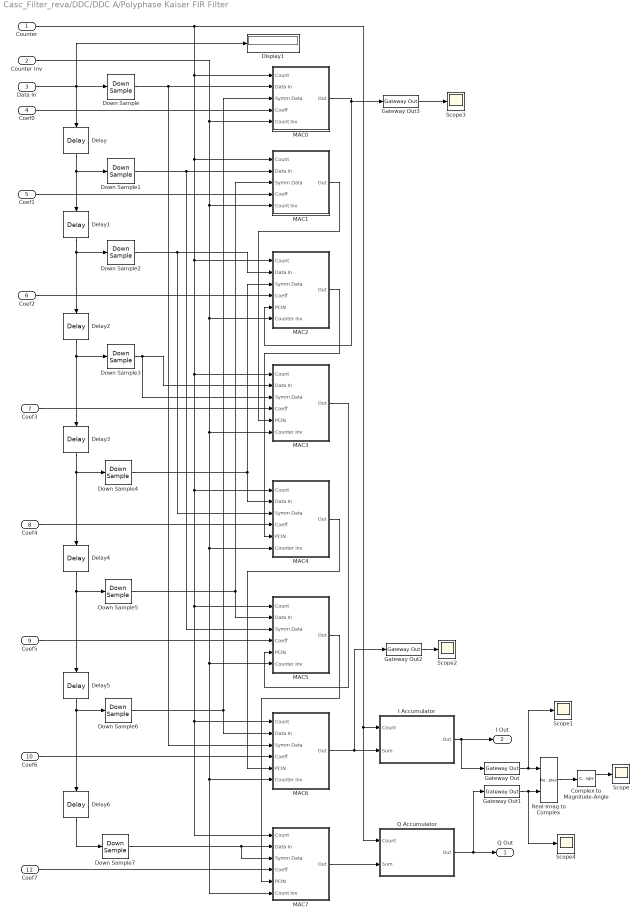
== system Casc_Filter_reva/DDC/DDC A/Polyphase Kaiser FIR Filter ==
  Counter : Inport
  Counter Inv : Inport  Port=2
  Data In : Inport  Port=3
  Coef0 : Inport  Port=4
  Coef1 : Inport  Port=5
  Coef2 : Inport  Port=6
  Coef3 : Inport  Port=7
  Coef4 : Inport  Port=8
  Coef5 : Inport  Port=9
  Coef6 : Inport  Port=10
  Coef7 : Inport  Port=11
  Complex to Magnitude-Angle : ComplexToMagnitudeAngle
  Delay{,1..6} (7 alike) : xbsIndex_r4/Delay  Orientation=down  en=off  latency=1  dbl_ovrd=off  reg_retiming=off  block_type=delay
      settings: infoedit=Hardware notes: A delay line is a chain, each link of which is an SRL16 followed by a flip-flop. If register retiming is enabled, the delay line is a chain of flip-flops.  block_version=8.2
  Display1 : Display
  Down Sample{,1..7} (8 alike) : xbsIndex_r4/Down Sample  sample_ratio=8  sample_phase="Last Value of Frame  (most efficient)"  en=off  latency=1  dbl_ovrd=off  block_type=dsamp
      settings: block_version=8.2
  Gateway Out{,1..3} (4 alike) : xbsIndex_r4/Gateway Out  hdl_port=off  timing_constraint=None  locs_specified=off  LOCs={}  block_type=gatewayout
      settings: infoedit="Gateway out block.  Converts Xilinx fixed point inputs into ouputs of type Simulink integer, double, or fixed point.<P><P>Hardware notes:  In hardware these blocks become top level output ports or are discarded, depending on how they are configured."  block_version=8.2
  I Accumulator : Subsystem
  MAC0 : Subsystem
  MAC1 : Subsystem
  MAC2 : Subsystem
  MAC3 : Subsystem
  MAC4 : Subsystem
  MAC5 : Subsystem
  MAC6 : Subsystem
  MAC7 : Subsystem
  Q Accumulator : Subsystem
  Real-Imag to Complex : RealImagToComplex
  Scope{,1..4} (5 alike) : Scope
      Scope2 settings: SaveName=ScopeData5
      Scope3 settings: SaveName=ScopeData6
      Scope4 settings: SaveName=ScopeData7
  Q Out : Outport
  I Out : Outport  Port=2
  wires:
  Coef7/1 -> MAC7/4(Coeff)
  Coef6/1 -> MAC6/4(Coeff)
  Coef5/1 -> MAC5/4(Coeff)
  Coef4/1 -> MAC4/4(Coeff)
  MAC5/1(Out) -> MAC7/5(PCIN)
  Down Sample7/1 -> MAC7/2(Data In), MAC7/3(Symm Data)
  MAC4/1(Out) -> MAC6/5(PCIN)
  Down Sample/1 -> MAC0/2(Data In), MAC6/3(Symm Data)
  Down Sample1/1 -> MAC1/2(Data In), MAC5/3(Symm Data)
  MAC3/1(Out) -> MAC5/5(PCIN)
  MAC2/1(Out) -> MAC4/5(PCIN)
  MAC1/1(Out) -> MAC3/5(PCIN)
  Down Sample3/1 -> MAC3/2(Data In), MAC3/3(Symm Data)
  Coef3/1 -> MAC3/4(Coeff)
  Coef2/1 -> MAC2/4(Coeff)
  MAC0/1(Out) -> MAC2/5(PCIN), Gateway Out3/1
  Down Sample2/1 -> MAC2/2(Data In), MAC4/3(Symm Data)
  Down Sample4/1 -> MAC2/3(Symm Data), MAC4/2(Data In)
  Down Sample5/1 -> MAC5/2(Data In), MAC1/3(Symm Data)
  Down Sample6/1 -> MAC0/3(Symm Data), MAC6/2(Data In)
  Delay6/1 -> Down Sample7/1
  Delay5/1 -> Down Sample6/1, Delay6/1
  Delay4/1 -> Down Sample5/1, Delay5/1
  Delay3/1 -> Down Sample4/1, Delay4/1
  Gateway Out1/1 -> Real-Imag to Complex/2, Scope4/1
  Gateway Out/1 -> Real-Imag to Complex/1, Scope1/1
  Complex to Magnitude-Angle/1 -> Scope/1
  Real-Imag to Complex/1 -> Complex to Magnitude-Angle/1
  Counter Inv/1 -> MAC1/5(Count Inv), MAC2/6(Counter Inv), MAC4/6(Counter Inv), MAC6/6(Counter Inv), MAC7/6(Count Inv), MAC5/6(Counter Inv), MAC3/6(Counter Inv), MAC0/5(Count Inv)
  MAC7/1(Out) -> Q Accumulator/2(Sum)
  MAC6/1(Out) -> I Accumulator/2(Sum), Gateway Out2/1
  Q Accumulator/1(Out) -> Q Out/1, Gateway Out1/1
  Counter/1 -> MAC1/1(Count), MAC2/1(Count), MAC3/1(Count), MAC4/1(Count), MAC7/1(Count), MAC6/1(Count), MAC5/1(Count), MAC0/1(Count), Q Accumulator/1(Count), I Accumulator/1(Count)
  I Accumulator/1(Out) -> I Out/1, Gateway Out/1
  Coef1/1 -> MAC1/4(Coeff)
  Coef0/1 -> MAC0/4(Coeff)
  Delay2/1 -> Down Sample3/1, Delay3/1
  Delay1/1 -> Down Sample2/1, Delay2/1
  Delay/1 -> Down Sample1/1, Delay1/1
  Data In/1 -> Down Sample/1, Delay/1, Display1/1
  Gateway Out2/1 -> Scope2/1
  Gateway Out3/1 -> Scope3/1

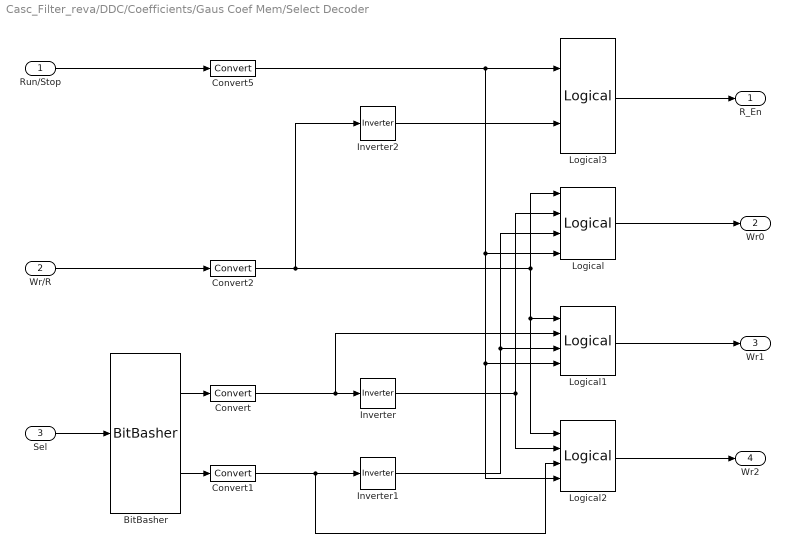
== system Casc_Filter_reva/DDC/Coefficients/Gaus Coef Mem/Select Decoder ==
  Run/Stop : Inport
  Wr/R : Inport  Port=2
  Sel : Inport  Port=3
  BitBasher : xbsIndex_r4/BitBasher  bitexpr=|  display_expr=off  sr_1=1  arith_type1=Unsigned  bin_pt1=0  sr_2=2  arith_type2=Unsigned  bin_pt2=0  sr_3=3  arith_type3=Unsigned  bin_pt3=0  sr_4=4  arith_type4=Unsigned  bin_pt4=0  dbl_ovrd=off  block_type=bitbasher
      | <html><head><meta name="qrichtext" content="1" /></head><body style="font-size:8pt;font-family:MS Shell Dlg">
      | <p>Sel0={Sel[0]}<br />Sel1={Sel[1]}<br /></p>
      | </body></html>
      settings: infoedit="Allows      extraction, concatenation and augmentation of bits"  block_version=VER_STRING_GOES_HERE
  Convert{,1..2,5} (4 alike) : xbsIndex_r4/Convert  arith_type=Boolean  n_bits=16  bin_pt=14  quantization=Truncate  overflow=Wrap  latency=0  dbl_ovrd=off  pipeline=off  block_type=convert
      settings: xl_area=[0 0 0 0 0 0 0]  block_version=VER_STRING_GOES_HERE
  Inverter : xbsIndex_r4/Inverter  en=off  latency=0  dbl_ovrd=off  block_type=inv
      settings: block_version=VER_STRING_GOES_HERE
  Inverter1 : xbsIndex_r4/Inverter  en=off  latency=0  dbl_ovrd=off  block_type=inv
      settings: block_version=VER_STRING_GOES_HERE
  Inverter2 : xbsIndex_r4/Inverter  en=off  latency=0  dbl_ovrd=off  block_type=inv
      settings: block_version=VER_STRING_GOES_HERE
  Logical : xbsIndex_r4/Logical  logical_function=AND  inputs=4  en=off  latency=0  precision=Full  arith_type=Unsigned  n_bits=16  bin_pt=0  align_bp=on  dbl_ovrd=off  block_type=logical
      settings: block_version=VER_STRING_GOES_HERE
  Logical1 : xbsIndex_r4/Logical  logical_function=AND  inputs=4  en=off  latency=0  precision=Full  arith_type=Unsigned  n_bits=16  bin_pt=0  align_bp=on  dbl_ovrd=off  block_type=logical
      settings: block_version=VER_STRING_GOES_HERE
  Logical2 : xbsIndex_r4/Logical  logical_function=AND  inputs=4  en=off  latency=0  precision=Full  arith_type=Unsigned  n_bits=16  bin_pt=0  align_bp=on  dbl_ovrd=off  block_type=logical
      settings: block_version=VER_STRING_GOES_HERE
  Logical3 : xbsIndex_r4/Logical  logical_function=AND  inputs=2  en=off  latency=0  precision=Full  arith_type=Unsigned  n_bits=16  bin_pt=0  align_bp=on  dbl_ovrd=off  block_type=logical
      settings: block_version=VER_STRING_GOES_HERE
  R_En : Outport
  Wr0 : Outport  Port=2
  Wr1 : Outport  Port=3
  Wr2 : Outport  Port=4
  wires:
  BitBasher/1 -> Convert/1
  BitBasher/2 -> Convert1/1
  Sel/1 -> BitBasher/1
  Logical/1 -> Wr0/1
  Logical1/1 -> Wr1/1
  Logical2/1 -> Wr2/1
  Wr/R/1 -> Convert2/1
  Convert/1 -> Inverter/1, Logical1/2
  Convert1/1 -> Inverter1/1, Logical2/3
  Convert2/1 -> Inverter2/1, Logical/1, Logical1/1, Logical2/1
  Inverter/1 -> Logical/2, Logical2/2
  Inverter1/1 -> Logical/3, Logical1/3
  Run/Stop/1 -> Convert5/1
  Convert5/1 -> Logical3/1, Logical/4, Logical1/4, Logical2/4
  Inverter2/1 -> Logical3/2
  Logical3/1 -> R_En/1

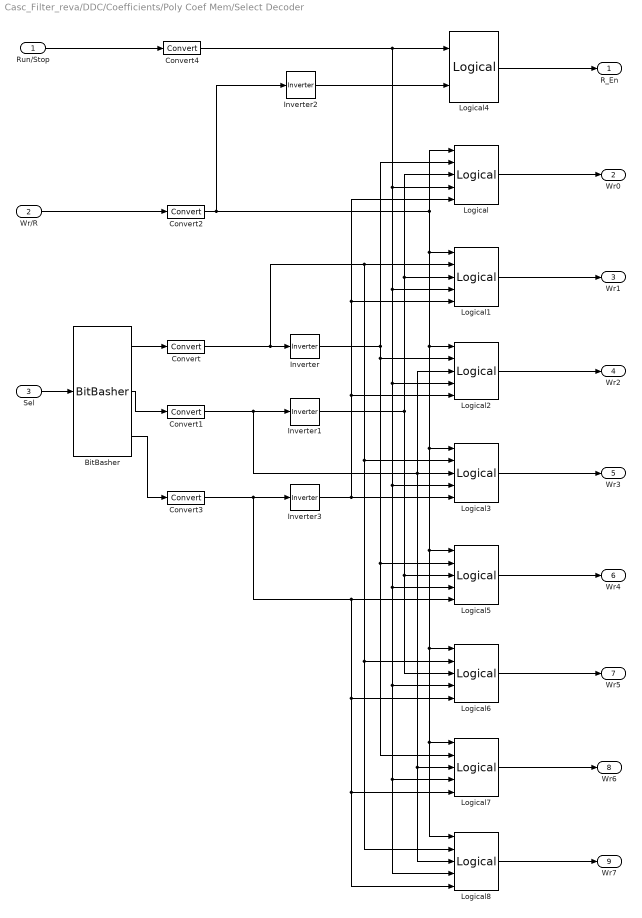
== system Casc_Filter_reva/DDC/Coefficients/Poly Coef Mem/Select Decoder ==
  Run/Stop : Inport
  Wr/R : Inport  Port=2
  Sel : Inport  Port=3
  BitBasher : xbsIndex_r4/BitBasher  bitexpr=|  display_expr=off  sr_1=1  arith_type1=Unsigned  bin_pt1=0  sr_2=2  arith_type2=Unsigned  bin_pt2=0  sr_3=3  arith_type3=Unsigned  bin_pt3=0  sr_4=4  arith_type4=Unsigned  bin_pt4=0  dbl_ovrd=off  block_type=bitbasher
      | <html><head><meta name="qrichtext" content="1" /><style type="text/css">
      | p, li { white-space: pre-wrap; }
      | </style></head><body style=" font-family:'MS Shell Dlg 2'; font-size:8.25pt; font-weight:400; font-style:normal;">
      | <p style=" margin-top:12px; margin-bottom:12px; margin-left:0px; margin-right:0px; -qt-block-indent:0; text-indent:0px; font-family:'MS Shell Dlg'; font-size:8pt;">Sel0={Sel[0]}<br />Sel1={Sel[1]}<br />Sel2={Sel[2]}</p></body></html>
      settings: infoedit="Allows      extraction, concatenation and augmentation of bits"  block_version=VER_STRING_GOES_HERE
  Convert{,1..4} (5 alike) : xbsIndex_r4/Convert  arith_type=Boolean  n_bits=16  bin_pt=14  quantization=Truncate  overflow=Wrap  latency=0  dbl_ovrd=off  pipeline=on  block_type=convert
      settings: xl_area=[0 0 0 0 0 0 0]  block_version=VER_STRING_GOES_HERE
  Inverter{,1..3} (4 alike) : xbsIndex_r4/Inverter  en=off  latency=0  dbl_ovrd=off  block_type=inv
      settings: block_version=VER_STRING_GOES_HERE
  Logical{,1..3,5..8} (8 alike) : xbsIndex_r4/Logical  logical_function=AND  inputs=5  en=off  latency=0  precision=Full  arith_type=Unsigned  n_bits=16  bin_pt=0  align_bp=on  dbl_ovrd=off  block_type=logical
      settings: block_version=VER_STRING_GOES_HERE
  Logical4 : xbsIndex_r4/Logical  logical_function=AND  inputs=2  en=off  latency=0  precision=Full  arith_type=Unsigned  n_bits=16  bin_pt=0  align_bp=on  dbl_ovrd=off  block_type=logical
      settings: block_version=VER_STRING_GOES_HERE
  R_En : Outport
  Wr0 : Outport  Port=2
  Wr1 : Outport  Port=3
  Wr2 : Outport  Port=4
  Wr3 : Outport  Port=5
  Wr4 : Outport  Port=6
  Wr5 : Outport  Port=7
  Wr6 : Outport  Port=8
  Wr7 : Outport  Port=9
  wires:
  BitBasher/1 -> Convert/1
  BitBasher/2 -> Convert1/1
  Sel/1 -> BitBasher/1
  Logical/1 -> Wr0/1
  Logical1/1 -> Wr1/1
  Logical2/1 -> Wr2/1
  Logical3/1 -> Wr3/1
  Wr/R/1 -> Convert2/1
  Convert/1 -> Inverter/1, Logical1/2, Logical3/2, Logical6/2, Logical8/2
  Convert1/1 -> Inverter1/1, Logical3/3, Logical2/3, Logical7/3, Logical8/3
  Convert2/1 -> Inverter2/1, Logical/1, Logical1/1, Logical2/1, Logical3/1, Logical5/1, Logical6/1, Logical7/1, Logical8/1
  Inverter/1 -> Logical/2, Logical2/2, Logical5/2, Logical7/2
  Inverter1/1 -> Logical/3, Logical1/3, Logical5/3, Logical6/3
  Run/Stop/1 -> Convert4/1
  Convert4/1 -> Logical4/1, Logical/4, Logical1/4, Logical2/4, Logical3/4, Logical5/4, Logical6/4, Logical7/4, Logical8/4
  Inverter2/1 -> Logical4/2
  Logical4/1 -> R_En/1
  BitBasher/3 -> Convert3/1
  Convert3/1 -> Inverter3/1, Logical5/5, Logical6/5, Logical7/5, Logical8/5
  Inverter3/1 -> Logical/5, Logical1/5, Logical2/5, Logical3/5
  Logical5/1 -> Wr4/1
  Logical6/1 -> Wr5/1
  Logical7/1 -> Wr6/1
  Logical8/1 -> Wr7/1

== system Casc_Filter_reva/DDC/DDC A/Gaussian FIR Filters/Gaussian FIR Filter ==
  Counter : Inport
  Counter Inv : Inport  Port=2
  Data In : Inport  Port=3
  Coef0 : Inport  Port=4
  Coef1 : Inport  Port=5
  Coef2 : Inport  Port=6
  Gaussian Accumulate : Subsystem
  Gaussian Mult : Subsystem
  Symmetric Data Flow : Subsystem
  Data Out : Outport
  wires:
  Counter/1 -> Gaussian Accumulate/1(Counter), Symmetric Data Flow/2(Counter)
  Gaussian Mult/1(Sum Out) -> Gaussian Accumulate/2(Data In)
  Symmetric Data Flow/1(Data 1) -> Gaussian Mult/1(Data 1)
  Symmetric Data Flow/2(Data 2) -> Gaussian Mult/2(Data 2)
  Data In/1 -> Symmetric Data Flow/1(Data In)
  Gaussian Accumulate/1(Data Out) -> Data Out/1
  Symmetric Data Flow/3(Data 3) -> Gaussian Mult/3(Data 3)
  Coef0/1 -> Gaussian Mult/4(Coeff 1)
  Coef1/1 -> Gaussian Mult/5(Coeff 2)
  Counter Inv/1 -> Symmetric Data Flow/3(Counter Inv)
  Coef2/1 -> Gaussian Mult/6(Coeff 3)

== system Casc_Filter_reva/DDC/DDC A/Gaussian FIR Filters/Gaussian FIR Filter1 ==
  Counter : Inport
  Counter Inv : Inport  Port=2
  Data In : Inport  Port=3
  Coef0 : Inport  Port=4
  Coef1 : Inport  Port=5
  Coef2 : Inport  Port=6
  Gaussian Accumulate : Subsystem
  Gaussian Mult : Subsystem
  Symmetric Data Flow : Subsystem
  Data Out : Outport
  wires:
  Counter/1 -> Gaussian Accumulate/1(Counter), Symmetric Data Flow/2(Counter)
  Gaussian Mult/1(Sum Out) -> Gaussian Accumulate/2(Data In)
  Symmetric Data Flow/1(Data 1) -> Gaussian Mult/1(Data 1)
  Symmetric Data Flow/2(Data 2) -> Gaussian Mult/2(Data 2)
  Data In/1 -> Symmetric Data Flow/1(Data In)
  Gaussian Accumulate/1(Data Out) -> Data Out/1
  Symmetric Data Flow/3(Data 3) -> Gaussian Mult/3(Data 3)
  Coef0/1 -> Gaussian Mult/4(Coeff 1)
  Coef1/1 -> Gaussian Mult/5(Coeff 2)
  Counter Inv/1 -> Symmetric Data Flow/3(Counter Inv)
  Coef2/1 -> Gaussian Mult/6(Coeff 3)

== system Casc_Filter_reva/DDC/DDC A/Polyphase Kaiser FIR Filter/I Accumulator ==
  Count : Inport
  Sum : Inport  Port=2
  Constant : xbsIndex_r4/Constant  arith_type=Signed (2's comp)  const=16383  n_bits=48  bin_pt=0  explicit_period=off  period=1  equ=P=C  opselect=C  inp2=PCIN>>17  opr=+  inp1=P  carry=CIN  dbl_ovrd=off  block_type=constant
      settings: block_version=8.2
  Constant1 : xbsIndex_r4/Constant  arith_type=Unsigned  const=0  n_bits=1  bin_pt=0  explicit_period=off  period=1  equ=P=C  opselect=C  inp2=PCIN>>17  opr=+  inp1=P  carry=CIN  dbl_ovrd=off  block_type=constant
      settings: block_version=8.2
  Constant6 : xbsIndex_r4/Constant  arith_type=Signed (2's comp)  const=0  n_bits=18  bin_pt=0  explicit_period=off  period=1  equ=P=PCIN+(A*B)  opselect=PCIN + A*B  inp2=PCIN>>17  opr=+  inp1=P  carry=CIN  dbl_ovrd=off  block_type=constant
      settings: block_version=8.2
  Constant7 : xbsIndex_r4/Constant  arith_type=Signed (2's comp)  const=0  n_bits=18  bin_pt=0  explicit_period=off  period=1  equ=P=PCIN+(A*B)  opselect=PCIN + A*B  inp2=PCIN>>17  opr=+  inp1=P  carry=CIN  dbl_ovrd=off  block_type=constant
      settings: block_version=8.2
  Constant8 : xbsIndex_r4/Constant  arith_type=DSP48 Instruction  const=1  n_bits=16  bin_pt=14  explicit_period=off  period=1  equ=P=PCIN+(P)  opselect=Custom  inp2=PCIN  opr=+  inp1=P  carry=0  dbl_ovrd=off  block_type=constant
      settings: block_version=8.2
  Constant9 : xbsIndex_r4/Constant  arith_type=DSP48 Instruction  const=1  n_bits=16  bin_pt=14  explicit_period=off  period=1  equ=P=PCIN+(C)  opselect=Custom  inp2=PCIN  opr=+  inp1=C  carry=0  dbl_ovrd=off  block_type=constant
      settings: block_version=8.2
  DSP2 : xbsIndex_r4/DSP48  use_b=Direct from B Port  use_op=on  use_creg=on  use_pcin=on  use_pcout=off  use_bcout=off  rst_all=off  en_all=off  pipeline_a=0  pipeline_b=0  pipeline_c=on  pipeline_p=on  pipeline_mult=off  pipeline_opmode=on  pipeline_sub=off  pipeline_carryin=off  pipeline_carryinsel=off  rst_a=off  rst_b=off  rst_c=off  rst_mult=off  rst_p=off  rst_carry_in=off  rst_ctrl=off  en_a=off  en_b=off  en_c=off  en_mult=off  en_p=off  en_carry_in=off  en_ctrl=off  dbl_ovrd=off  use_synth_model=off  xl_useadderonly=on  block_type=dsp48
      settings: block_version=8.2
  Delay : xbsIndex_r4/Delay  en=off  latency=2  dbl_ovrd=off  reg_retiming=off  block_type=delay
      settings: infoedit=Hardware notes: A delay line is a chain, each link of which is an SRL16 followed by a flip-flop. If register retiming is enabled, the delay line is a chain of flip-flops.  block_version=8.2
  Down Sample1 : xbsIndex_r4/Down Sample  sample_ratio=downsample  sample_phase="Last Value of Frame  (most efficient)"  en=off  latency=1  dbl_ovrd=off  block_type=dsamp
      settings: block_version=8.2
  Mux : xbsIndex_r4/Mux  inputs=2  en=off  latency=1  precision=Full  arith_type=Unsigned  n_bits=16  bin_pt=14  quantization=Truncate  overflow=Wrap  dbl_ovrd=off  block_type=mux
      settings: block_version=8.2
  Register : xbsIndex_r4/Register  init=0  rst=off  en=off  dbl_ovrd=off  block_type=register
      settings: block_version=8.2
  Register1 : xbsIndex_r4/Register  Orientation=down  init=0  rst=off  en=on  dbl_ovrd=off  block_type=register
      settings: block_version=8.2
  Reinterpret : xbsIndex_r4/Reinterpret  force_arith_type=on  arith_type="Signed  (2's comp)"  force_bin_pt=on  bin_pt=17  block_type=reinterpret
      settings: infoedit="Changes signal type without altering the binary representation.   You can changed the signal between signed and unsigned, and relocate the binary point.<P><P>Hardware notes: In hardware this block costs nothing.<P><P>Example:  Suppose the input is 6 bits wide, signed, with 2 fractional bits, and the output is forced to unsigned with 0 fractional bits.  Then an input of -2.0 (1110.00 in binary 2's complement) becomes an output of 56 (111000 in binary)."  block_version=8.2
  Relational : xbsIndex_r4/Relational  mode=a=b  en=off  latency=6  dbl_ovrd=off  block_type=relational
      settings: block_version=8.2
  Slice : xbsIndex_r4/Slice  nbits=16  boolean_output=off  mode=Two Bit Locations  bit1=-15  base1=MSB of Input  bit0=15  base0=LSB of Input  dbl_ovrd=off  block_type=slice
      settings: infoedit="Extracts a given range of bits from each input sample and presents it at the output.  The output type is ordinarily unsigned with binary point at zero, but can be Boolean when the slice is one bit wide.<P><P>Hardware notes: In hardware this block costs nothing."  block_version=8.2
  Out : Outport
  wires:
  Register1/1 -> Down Sample1/1
  Constant1/1 -> Relational/2
  Count/1 -> Relational/1
  Relational/1 -> Mux/1, Delay/1
  Reinterpret/1 -> Register/1
  Constant6/1 -> DSP2/1
  Constant7/1 -> DSP2/2
  DSP2/1 -> Register1/1
  Constant9/1 -> Mux/3
  Constant8/1 -> Mux/2
  Delay/1 -> Register1/2
  Slice/1 -> Reinterpret/1
  Register/1 -> Out/1
  Mux/1 -> DSP2/5
  Sum/1 -> DSP2/4
  Constant/1 -> DSP2/3
  Down Sample1/1 -> Slice/1
